simulink subsystem "dummyNav"  (R2026a)
settings: Solver=VariableStepAuto
settings Model: Creator=maxhu  LastModifiedBy=maxhu

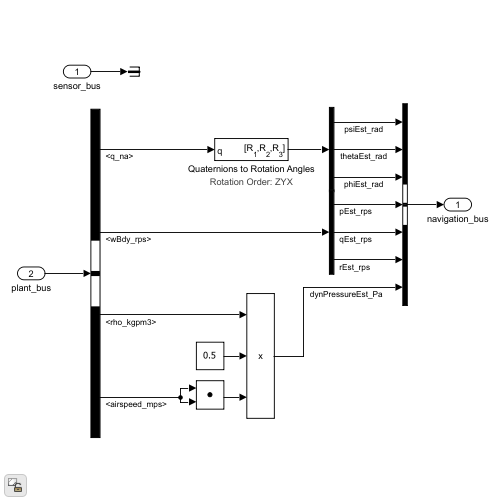
[thumbnail: Simulink's stored preview of the top-level diagram]
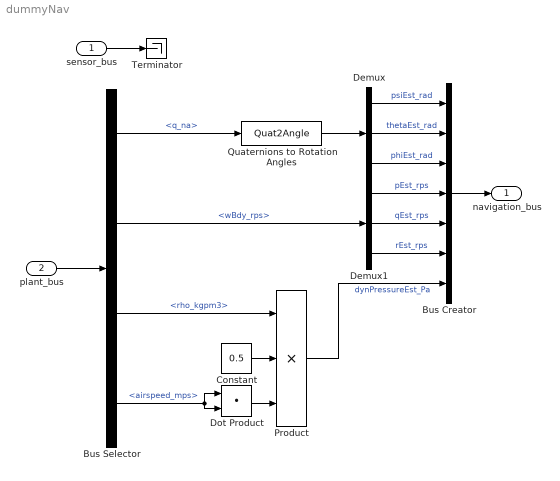
== system dummyNav ==
  sensor_bus : Inport
  plant_bus : Inport  Port=2
  Bus Creator : BusCreator  Inputs=7
  Bus Selector : BusSelector  OutputSignals=eom_bus.q_na,eom_bus.wBdy_rps,enviroment_bus.rho_kgpm3,enviroment_bus.airspeed_mps
  Constant : Constant  Value=0.5
  Demux : Demux  Outputs=3
  Demux1 : Demux  Outputs=3
  Dot Product : DotProduct  OutDataTypeStr=Inherit: Inherit via internal rule
  Product : Product  Inputs=3
  Quaternions to Rotation Angles : Quat2Angle
      settings: AttributesFormatString=Rotation Order: %<rotationOrder>
  Terminator : Terminator
  navigation_bus : Outport
  wires:
  sensor_bus/1 -> Terminator/1
  Bus Creator/1 -> navigation_bus/1
  Demux/1 -> Bus Creator/1  "psiEst_rad"
  Demux/2 -> Bus Creator/2  "thetaEst_rad"
  Demux/3 -> Bus Creator/3  "phiEst_rad"
  Demux1/2 -> Bus Creator/5  "qEst_rps"
  Demux1/1 -> Bus Creator/4  "pEst_rps"
  Demux1/3 -> Bus Creator/6  "rEst_rps"
  Quaternions to Rotation Angles/1 -> Demux/1
  Product/1 -> Bus Creator/7  "dynPressureEst_Pa"
  Dot Product/1 -> Product/3
  Bus Selector/1 -> Quaternions to Rotation Angles/1  "<q_na>"
  plant_bus/1 -> Bus Selector/1
  Bus Selector/3 -> Product/1  "<rho_kgpm3>"
  Bus Selector/2 -> Demux1/1  "<wBdy_rps>"
  Bus Selector/4 -> Dot Product/2, Dot Product/1  "<airspeed_mps>"
  Constant/1 -> Product/2
